simulink model "eZdsp_Test"  (R2020a)
settings: Solver=FixedStepDiscrete  StartTime=0.0  StopTime=inf  FixedStep=T  RelTol=1e-3  EnableMultiTasking=on
undefined symbols (not defined in the file): ILmax, Iumax, T, Ucmax, wmax
libraries: c280xlib x9, simulink x4, c2833xlib x1
settings Model: ExtModeTrigDuration=8  Creator=Nguyen Tung  LastModifiedBy=Nguyen Tung
settings OptimizationCC: DefaultUnderspecifiedDataType=single  StrengthReduction=on  PassReuseOutputArgsAs=Individual arguments  MaxStackSize=1024  OptimizeBlockOrder=speed  OptimizationPriority=Speed  OptimizationCustomize=off  MultiThreadedLoops=on  DenormalBehavior=FlushToZero  EfficientTunableParamExpr=on
settings DebuggingCC: ParameterTunabilityLossMsg=error
settings HardwareCC: ProdBitPerChar=16  ProdBitPerInt=16  ProdBitPerPointer=32  ProdBitPerSizeT=32  ProdBitPerPtrDiffT=32  ProdLargestAtomicInteger=Integer  ProdLargestAtomicFloat=None  ProdWordSize=16  ProdLongLongMode=on  ProdHWDeviceType=Texas Instruments->C2000
settings SFSimCC: MATLABDynamicMemAlloc=off
settings RTWCC: SystemTargetFile=ert.tlc  HardwareBoard=TI Delfino F2833x  TLCOptions=-aInlineSetEventsForThisBaseRateFcn=TLC_FALSE -aSuppressMultiTaskScheduler=TLC_FALSE -aRateBasedStepFcn=1  TemplateMakefile=ert_default_tmf  GenerateReport=on  Toolchain=Texas Instruments Code Composer Studio (C2000)
settings CodeAppCC: ForceParamTrailComments=on  IgnoreCustomStorageClasses=off  OperatorAnnotations=on  SimulinkDataObjDesc=on  SFDataObjDesc=on  InsertBlockDesc=on
settings ERTTargetCC: CodeReplacementLibrary=TI C28x  ExtModeStaticAllocSize=10000

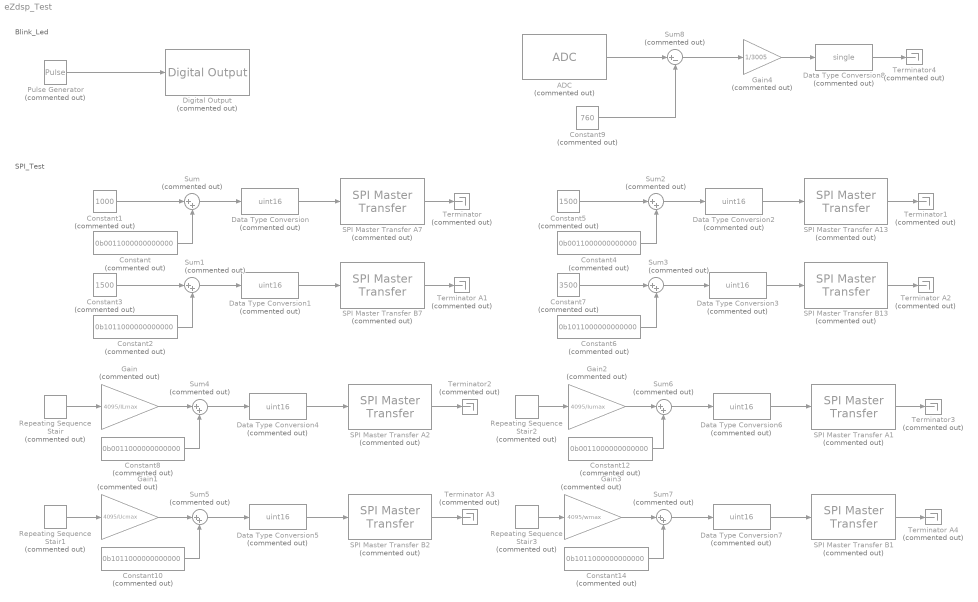
== system eZdsp_Test ==
  note: SPI_Test
  note: Blink_Led
  ADC : c280xlib/ADC  Commented=on  useModule=A  useMode=Sequential  sourceSOC=Software  sourceSOC1=Software  sourceSOC2=ePWMxB  xint2_ADCSOC=31  Ts=T  dType=uint16  postInterrupt=off  numConversionsSingle=1  numConversionsDouble=1  conv0=ADCINA0  conv1=ADCINA1  conv2=ADCINA2  conv3=ADCINA3  conv4=ADCINA4  conv5=ADCINA5  conv6=ADCINA6  conv7=ADCINA7  conv8=ADCINB0  conv9=ADCINB1  conv10=ADCINB2  conv11=ADCINB3  conv12=ADCINB4  conv13=ADCINB5  conv14=ADCINB6  conv15=ADCINB7  convAB0=ADCINA0 and ADCINB0  convAB1=ADCINA1 and ADCINB1  convAB2=ADCINA2 and ADCINB2  convAB3=ADCINA3 and ADCINB3  convAB4=ADCINA4 and ADCINB4  convAB5=ADCINA5 and ADCINB5  convAB6=ADCINA6 and ADCINB6  convAB7=ADCINA7 and ADCINB7  convA0=ADCINA0  convA1=ADCINA1  convA2=ADCINA2  convA3=ADCINA3  convA4=ADCINA4  convA5=ADCINA5  convA6=ADCINA6  convA7=ADCINA7  convB0=ADCINB0  convB1=ADCINB1  convB2=ADCINB2  convB3=ADCINB3  convB4=ADCINB4  convB5=ADCINB5  convB6=ADCINB6  convB7=ADCINB7  c28xmultiPort=off  endma=off  chdma=1
      settings: SourceProductBaseCode=TIC2000
  Constant{,4,8,12} (4 alike) : Constant  Commented=on  Value=0b0011000000000000
  Constant1 : Constant  Commented=on  Value=1000
  Constant{2,6,10,14} (4 alike) : Constant  Commented=on  Value=0b1011000000000000
  Constant3 : Constant  Commented=on  Value=1500
  Constant5 : Constant  Commented=on  Value=1500
  Constant7 : Constant  Commented=on  Value=3500
  Constant9 : Constant  Commented=on  Value=760
  Data Type Conversion{,1..7} (8 alike) : DataTypeConversion  Commented=on  OutDataTypeStr=uint16
  Data Type Conversion8 : DataTypeConversion  Commented=on  OutMin=[0]  OutMax=[1]  OutDataTypeStr=single  SaturateOnIntegerOverflow=on
  Digital Output : c2833xlib/Digital Output  Commented=on  GPIO_Number=GPIO32~GPIO39  GPIO_Bit0=on  GPIO_BIT0_Toggle=off  GPIO_Bit1=off  GPIO_BIT1_Toggle=off  GPIO_Bit2=off  GPIO_BIT2_Toggle=off  GPIO_Bit3=off  GPIO_BIT3_Toggle=off  GPIO_Bit4=off  GPIO_BIT4_Toggle=off  GPIO_Bit5=off  GPIO_BIT5_Toggle=off  GPIO_Bit6=off  GPIO_BIT6_Toggle=off  GPIO_Bit7=off  GPIO_BIT7_Toggle=off
      settings: SourceProductBaseCode=TIC2000
  Gain : Gain  Commented=on  Gain=4095/ILmax
  Gain1 : Gain  Commented=on  Gain=4095/Ucmax
  Gain2 : Gain  Commented=on  Gain=4095/Iumax
  Gain3 : Gain  Commented=on  Gain=4095/wmax
  Gain4 : Gain  Commented=on  Gain=1/3005
  Pulse Generator : DiscretePulseGenerator  Commented=on  PulseType=Time based  Period=1  PulseWidth=50
  Repeating Sequence Stair : simulink/Sources/Repeating Sequence Stair  Commented=on  OutValues=[0 10 20 30 40 50 60].'  tsamp=T  OutMin=[]  OutMax=[]  OutDataTypeStr=double  OutputDataTypeScalingMode=double  OutDataType=fixdt(0,8)  ConRadixGroup=Best Precision: Vector-wise  OutScaling=2^-12
  Repeating Sequence Stair1 : simulink/Sources/Repeating Sequence Stair  Commented=on  OutValues=[0 50 100 150 200 250 300 350 400].'  tsamp=T  OutMin=[]  OutMax=[]  OutDataTypeStr=double  OutputDataTypeScalingMode=double  OutDataType=fixdt(0,8)  ConRadixGroup=Best Precision: Vector-wise  OutScaling=2^-12
  Repeating Sequence Stair2 : simulink/Sources/Repeating Sequence Stair  Commented=on  OutValues=[0 10 20 30 40 50 60].'  tsamp=T  OutMin=[]  OutMax=[]  OutDataTypeStr=double  OutputDataTypeScalingMode=double  OutDataType=fixdt(0,8)  ConRadixGroup=Best Precision: Vector-wise  OutScaling=2^-12
  Repeating Sequence Stair3 : simulink/Sources/Repeating Sequence Stair  Commented=on  OutValues=[0 10 20 30 40 50 60 70 80 90 100].'  tsamp=T  OutMin=[]  OutMax=[]  OutDataTypeStr=double  OutputDataTypeScalingMode=double  OutDataType=fixdt(0,8)  ConRadixGroup=Best Precision: Vector-wise  OutScaling=2^-12
  SPI Master Transfer A1 : c280xlib/SPI Master Transfer  Commented=on  SPISelect=SPI_A  ClockPolarity=Falling_edge  ClockPhase=No_delay  SPIModule=uint32(0)  Mode=Master  BusSpeed=uint32(1000000)  FirstBitToTransfer=Most significant bit (MSB)  ClockMode=0  BlockFunction=Transfer  EnableRegisterAddress=off  RegisterAddress=0  OutputDataType=int8  OutputDataLength=1  DataBits=16  UseCustomSSPin=Explicit GPIO calls  ActiveLowSSPin=Active low  Pin=13
      settings: SourceProductBaseCode=TIC2000
  SPI Master Transfer A13 : c280xlib/SPI Master Transfer  Commented=on  SPISelect=SPI_A  ClockPolarity=Falling_edge  ClockPhase=No_delay  SPIModule=uint32(0)  Mode=Master  BusSpeed=uint32(1000000)  FirstBitToTransfer=Most significant bit (MSB)  ClockMode=0  BlockFunction=Transfer  EnableRegisterAddress=off  RegisterAddress=0  OutputDataType=int8  OutputDataLength=1  DataBits=16  UseCustomSSPin=Explicit GPIO calls  ActiveLowSSPin=Active low  Pin=13
      settings: SourceProductBaseCode=TIC2000
  SPI Master Transfer A2 : c280xlib/SPI Master Transfer  Commented=on  SPISelect=SPI_A  ClockPolarity=Falling_edge  ClockPhase=No_delay  SPIModule=uint32(0)  Mode=Master  BusSpeed=uint32(1000000)  FirstBitToTransfer=Most significant bit (MSB)  ClockMode=0  BlockFunction=Transfer  EnableRegisterAddress=off  RegisterAddress=0  OutputDataType=int8  OutputDataLength=1  DataBits=16  UseCustomSSPin=Explicit GPIO calls  ActiveLowSSPin=Active low  Pin=7
      settings: SourceProductBaseCode=TIC2000
  SPI Master Transfer A7 : c280xlib/SPI Master Transfer  Commented=on  SPISelect=SPI_A  ClockPolarity=Falling_edge  ClockPhase=No_delay  SPIModule=uint32(0)  Mode=Master  BusSpeed=uint32(1000000)  FirstBitToTransfer=Most significant bit (MSB)  ClockMode=0  BlockFunction=Transfer  EnableRegisterAddress=off  RegisterAddress=0  OutputDataType=int8  OutputDataLength=1  DataBits=16  UseCustomSSPin=Explicit GPIO calls  ActiveLowSSPin=Active low  Pin=7
      settings: SourceProductBaseCode=TIC2000
  SPI Master Transfer B1 : c280xlib/SPI Master Transfer  Commented=on  SPISelect=SPI_A  ClockPolarity=Falling_edge  ClockPhase=No_delay  SPIModule=uint32(0)  Mode=Master  BusSpeed=uint32(1000000)  FirstBitToTransfer=Most significant bit (MSB)  ClockMode=0  BlockFunction=Transfer  EnableRegisterAddress=off  RegisterAddress=0  OutputDataType=int8  OutputDataLength=1  DataBits=16  UseCustomSSPin=Explicit GPIO calls  ActiveLowSSPin=Active low  Pin=13
      settings: SourceProductBaseCode=TIC2000
  SPI Master Transfer B13 : c280xlib/SPI Master Transfer  Commented=on  SPISelect=SPI_A  ClockPolarity=Falling_edge  ClockPhase=No_delay  SPIModule=uint32(0)  Mode=Master  BusSpeed=uint32(1000000)  FirstBitToTransfer=Most significant bit (MSB)  ClockMode=0  BlockFunction=Transfer  EnableRegisterAddress=off  RegisterAddress=0  OutputDataType=int8  OutputDataLength=1  DataBits=16  UseCustomSSPin=Explicit GPIO calls  ActiveLowSSPin=Active low  Pin=13
      settings: SourceProductBaseCode=TIC2000
  SPI Master Transfer B2 : c280xlib/SPI Master Transfer  Commented=on  SPISelect=SPI_A  ClockPolarity=Falling_edge  ClockPhase=No_delay  SPIModule=uint32(0)  Mode=Master  BusSpeed=uint32(1000000)  FirstBitToTransfer=Most significant bit (MSB)  ClockMode=0  BlockFunction=Transfer  EnableRegisterAddress=off  RegisterAddress=0  OutputDataType=int8  OutputDataLength=1  DataBits=16  UseCustomSSPin=Explicit GPIO calls  ActiveLowSSPin=Active low  Pin=7
      settings: SourceProductBaseCode=TIC2000
  SPI Master Transfer B7 : c280xlib/SPI Master Transfer  Commented=on  SPISelect=SPI_A  ClockPolarity=Falling_edge  ClockPhase=No_delay  SPIModule=uint32(0)  Mode=Master  BusSpeed=uint32(1000000)  FirstBitToTransfer=Most significant bit (MSB)  ClockMode=0  BlockFunction=Transfer  EnableRegisterAddress=off  RegisterAddress=0  OutputDataType=int8  OutputDataLength=1  DataBits=16  UseCustomSSPin=Explicit GPIO calls  ActiveLowSSPin=Active low  Pin=7
      settings: SourceProductBaseCode=TIC2000
  Sum{,1..7} (8 alike) : Sum  Commented=on  Inputs=|++
  Sum8 : Sum  Commented=on  Inputs=|+-
  Terminator{,1..4} (5 alike) : Terminator  Commented=on
  Terminator A{1..4} (4 alike) : Terminator  Commented=on
  wires:
  Pulse Generator/1 -> Digital Output/1
  SPI Master Transfer A7/1 -> Terminator/1
  Data Type Conversion/1 -> SPI Master Transfer A7/1
  Sum/1 -> Data Type Conversion/1
  Constant/1 -> Sum/2
  Constant1/1 -> Sum/1
  Constant3/1 -> Sum1/1
  Constant2/1 -> Sum1/2
  Sum1/1 -> Data Type Conversion1/1
  Data Type Conversion1/1 -> SPI Master Transfer B7/1
  SPI Master Transfer B7/1 -> Terminator A1/1
  Sum2/1 -> Data Type Conversion2/1
  Constant4/1 -> Sum2/2
  Constant6/1 -> Sum3/2
  SPI Master Transfer B13/1 -> Terminator A2/1
  Sum3/1 -> Data Type Conversion3/1
  Constant7/1 -> Sum3/1
  Data Type Conversion2/1 -> SPI Master Transfer A13/1
  Data Type Conversion3/1 -> SPI Master Transfer B13/1
  SPI Master Transfer A13/1 -> Terminator1/1
  Constant5/1 -> Sum2/1
  Gain2/1 -> Sum6/1
  SPI Master Transfer A1/1 -> Terminator3/1
  Data Type Conversion7/1 -> SPI Master Transfer B1/1
  Data Type Conversion6/1 -> SPI Master Transfer A1/1
  Gain3/1 -> Sum7/1
  Sum7/1 -> Data Type Conversion7/1
  SPI Master Transfer B1/1 -> Terminator A4/1
  Constant14/1 -> Sum7/2
  Constant12/1 -> Sum6/2
  Sum6/1 -> Data Type Conversion6/1
  SPI Master Transfer B2/1 -> Terminator A3/1
  Data Type Conversion5/1 -> SPI Master Transfer B2/1
  Sum5/1 -> Data Type Conversion5/1
  Constant10/1 -> Sum5/2
  Repeating Sequence Stair1/1 -> Gain1/1
  Repeating Sequence Stair/1 -> Gain/1
  Constant8/1 -> Sum4/2
  Sum4/1 -> Data Type Conversion4/1
  Data Type Conversion4/1 -> SPI Master Transfer A2/1
  SPI Master Transfer A2/1 -> Terminator2/1
  Gain/1 -> Sum4/1
  Gain1/1 -> Sum5/1
  Repeating Sequence Stair2/1 -> Gain2/1
  Repeating Sequence Stair3/1 -> Gain3/1
  ADC/1 -> Sum8/1
  Sum8/1 -> Gain4/1
  Constant9/1 -> Sum8/2
  Data Type Conversion8/1 -> Terminator4/1
  Gain4/1 -> Data Type Conversion8/1
